simulink model "Multiuav"  (Simulink 4.00)
settings: Solver=FixedStepDiscrete  StartTime=0.0  StopTime=g_StopTime  FixedStep=g_SampleTime  RelTol=1e-3
undefined symbols (not defined in the file): ATRFunctions, g_AssignmentAlgorithm, g_CommandTurnRadius, g_CoordinationDelayDen, g_DefaultWaypointAltitude, g_EnableTarget, g_EnableVehicle, g_EntityTypes, g_MaxNumberTargets, g_MaxNumberVehicles, g_MaxReassignmentDeltaTime, g_ObjectMessageIDs, g_OptionSaveDataAVDS, g_OptionSaveDataPlot, g_SampleTime, g_SensorRollLimitDeg, g_TargetStates, g_Tasks, g_TypeAssignment, g_VehicleInputFiles, g_VehicleMemory, g_VehicleTypes, g_WaypointDefinitions, g_WaypointTypes
libraries: cooperative x42
(part 3 of 4)

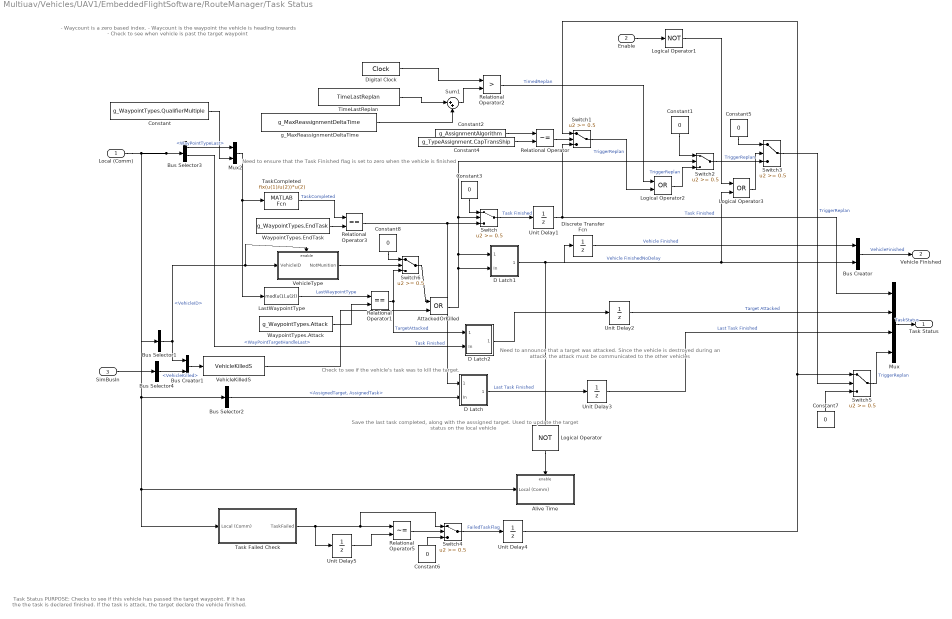
== system Multiuav/Vehicles/UAV1/EmbeddedFlightSoftware/RouteManager/Task Status ==
  note: - Waycount is a zero based index.
      | - Waycount is the waypoint the vehicle is
      | heading towards
      | - Check to see when vehicle is past the
      | target waypoint
  note: Need to ensure that the Task Finished
      | flag is set to zero when the vehicle is finished
  note: Check to see if the vehicle's
      | task was to kill the target.
  note: Need to announce that a target was
      | attacked. Since the vehicle is destroyed
      | during an attack, the attack must be
      | communicated to the other vehicles
  note: Save the last task completed,
      | along with the asssigned target.
      | Used to update the target status
      | on the local vehicle
  note: Task Status
      |
      | PURPOSE: Checks to see if this vehicle has passed the target waypoint. If it
      | has the the task is declared finished. If the task is attack, the target declare the
      | vehicle finished.
  Local (Comm) : Inport  Port=1  LatchInput=off  SampleTime=g_SampleTime
  Enable : Inport  Port=2  LatchInput=off  SampleTime=g_SampleTime
  SimBusIn : Inport  Port=3  LatchInput=off  SampleTime=g_SampleTime
  Alive Time : Subsystem  TreatAsAtomicUnit=on
      settings: RTWFcnNameOpts=Auto  RTWFileNameOpts=Auto
  AttackedOrKilled : Logic  Operator=OR  Inputs=2
  Bus Creator : BusCreator  Inputs=2
  Bus Creator1 : BusCreator  Inputs=2
  Bus Selector1 : BusSelector  OutputSignals=VehicleID  MuxedOutput=on
  Bus Selector2 : BusSelector  OutputSignals=Dynamics(com).TacticalManuevering.AssignedTarget,Dynamics(com).TacticalManuevering.AssignedTask  MuxedOutput=on
  Bus Selector3 : BusSelector  OutputSignals=Dynamics(com).TacticalManuevering.WayPointTypeLast,Dynamics(com).TacticalManuevering.WayPointTargetHandleLast  MuxedOutput=off
  Bus Selector4 : BusSelector  OutputSignals=ExternalTruth.VehicleKilled  MuxedOutput=on
  Constant : Constant  Value=g_WaypointTypes.QualifierMultiple
  Constant{1,3,5,8} (4 alike) : Constant  Orientation=down  Value=0
  Constant2 : Constant  Value=g_AssignmentAlgorithm
  Constant4 : Constant  Value=g_TypeAssignment.CapTransShip
  Constant6 : Constant  Orientation=up  Value=0
  Constant7 : Constant  Orientation=up  Value=0
  D Latch : Subsystem
      settings: RTWFcnNameOpts=Auto  RTWFileNameOpts=Auto
      mask Type: DLatch
      mask Description: D Latch Flip Flop Block
  D Latch1 : Subsystem
      settings: RTWFcnNameOpts=Auto  RTWFileNameOpts=Auto
      mask Type: DLatch
      mask Description: D Latch Flip Flop Block
  D Latch2 : Subsystem
      settings: RTWFcnNameOpts=Auto  RTWFileNameOpts=Auto
      mask Type: DLatch
      mask Description: D Latch Flip Flop Block
  Digital Clock : DigitalClock  SampleTime=g_SampleTime
  Discrete Transfer Fcn : DiscreteTransferFcn  Numerator=[1]  Denominator=[1 0 ]  SampleTime=g_SampleTime  Realization=auto
      settings: RTWStateStorageClass=Auto
  LastWaypointType : MATLABFcn  MATLABFcn=mod(u(1),u(2))  OutputDimensions=-1  OutputSignalType=auto  Output1D=on
  Logical Operator : Logic  Orientation=down  Operator=NOT  Inputs=2
  Logical Operator1 : Logic  Operator=NOT  Inputs=2
  Logical Operator2 : Logic  Operator=OR  Inputs=2
  Logical Operator3 : Logic  Operator=OR  Inputs=2
  Mux : Mux  Inputs=[1 1 2 1]
  Mux2 : Mux  Inputs=2
  Relational Operator : RelationalOperator  Operator=~=
  Relational Operator1 : RelationalOperator  Operator===
  Relational Operator2 : RelationalOperator  Operator=>
  Relational Operator3 : RelationalOperator  Operator===
  Relational Operator5 : RelationalOperator  Operator=~=
  Sum1 : Sum  Inputs=|++  SaturateOnIntegerOverflow=on
  Switch{,1..6} (7 alike) : Switch  Threshold=0.5
  Task Failed Check : Subsystem  TreatAsAtomicUnit=on
      settings: RTWFcnNameOpts=Auto  RTWFileNameOpts=Auto
  TaskCompleted : MATLABFcn  MATLABFcn=fix(u(1)/u(2))*u(2)  OutputDimensions=-1  OutputSignalType=auto  Output1D=on
  TimeLastReplan : DataStoreRead  DataStoreName=TimeLastReplan  SampleTime=g_SampleTime
  Unit Delay{1..5} (5 alike) : UnitDelay  X0=0  SampleTime=g_SampleTime
      settings: RTWStateStorageClass=Auto
  VehicleKilledS : S-Function  FunctionName=VehicleKilledS  Parameters=g_MaxNumberVehicles, g_MaxNumberTargets  PortCounts=[]  SFunctionModules=''
  VehicleType : Subsystem  TreatAsAtomicUnit=on
      settings: RTWFcnNameOpts=Auto  RTWFileNameOpts=Auto
  WaypointTypes.Attack : Constant  Value=g_WaypointTypes.Attack
  WaypointTypes.EndTask : Constant  Value=g_WaypointTypes.EndTask
  g_MaxReassignmentDeltaTime : Constant  Value=g_MaxReassignmentDeltaTime
  Task Status : Outport  Port=1
  Vehicle Finished : Outport  Port=2
  wires:
  Constant7/1 -> Switch5/3
  Switch5/1 -> Mux/4  "TriggerReplan"
  Unit Delay4/1 -> Switch5/1, Switch1/1
  Relational Operator2/1 -> Logical Operator2/1  "TimedReplan"
  Constant6/1 -> Switch4/3
  Switch4/1 -> Unit Delay4/1  "FailedTaskFlag"
  Unit Delay5/1 -> Relational Operator5/2
  Task Failed Check/1(TaskFailed) -> Switch4/1, Relational Operator5/1, Unit Delay5/1
  Local (Comm)/1 -> Task Failed Check/1(Local (Comm)), Alive Time/1(Local (Comm)), Bus Selector2/1, Bus Selector1/1, Bus Selector3/1
  WaypointTypes.EndTask/1 -> Relational Operator3/2
  WaypointTypes.Attack/1 -> Relational Operator1/2
  Constant3/1 -> Switch/1
  Switch/1 -> Unit Delay1/1  "Task Finished"
  Bus Selector2/1 -> D Latch/2(In)  "<AssignedTarget, AssignedTask>"
  Relational Operator3/1 -> D Latch/1(Enable), Switch/3  "Task Finished"
  Mux/1 -> Task Status/1  "TaskStatus"
  D Latch/1(Latched) -> Unit Delay3/1  "Last Task Finished"
  Discrete Transfer Fcn/1 -> Bus Creator/1  "Vehicle Finished"
  Unit Delay1/1 -> Switch1/3, Mux/1  "Task Finished"
  Unit Delay2/1 -> Mux/2  "Target Attacked"
  D Latch1/1(Latched) -> Discrete Transfer Fcn/1, Logical Operator/1, Bus Creator/2, Logical Operator3/2  "Vehicle FinishedNoDelay"
  Unit Delay3/1 -> Mux/3  "Last Task Finished"
  Bus Creator/1 -> Vehicle Finished/1  "VehicleFinished"
  Constant1/1 -> Switch2/1
  Logical Operator2/1 -> Switch2/3  "TriggerReplan"
  Bus Selector3/1 -> Mux2/1  "<WayPointTypeLast>"
  LastWaypointType/1 -> Relational Operator1/1  "LastWaypointType"
  TaskCompleted/1 -> Relational Operator3/1  "TaskCompleted"
  Constant/1 -> Mux2/2
  Mux2/1 -> LastWaypointType/1, TaskCompleted/1
  Bus Selector3/2 -> D Latch2/2(In)  "<WayPointTargetHandleLast>"
  D Latch2/1(Latched) -> Unit Delay2/1
  Logical Operator/1 -> Alive Time/Enable
  Relational Operator/1 -> Switch1/2
  Constant2/1 -> Relational Operator/1
  Constant4/1 -> Relational Operator/2
  Switch1/1 -> Logical Operator2/2  "TriggerReplan"
  Switch2/1 -> Switch3/3  "TriggerReplan"
  Relational Operator5/1 -> Switch4/2
  Sum1/1 -> Relational Operator2/2
  g_MaxReassignmentDeltaTime/1 -> Sum1/2
  TimeLastReplan/1 -> Sum1/1
  Digital Clock/1 -> Relational Operator2/1
  Constant5/1 -> Switch3/1
  Switch3/1 -> Switch5/2  "TriggerReplan"
  Logical Operator1/1 -> Logical Operator3/1
  Enable/1 -> Logical Operator1/1
  Logical Operator3/1 -> Switch3/2
  Bus Selector1/1 -> Bus Creator1/1, VehicleType/1(VehicleID), VehicleType/Enable  "<VehicleID>"
  Relational Operator1/1 -> Switch6/3, D Latch2/1(Enable)  "TargetAttacked"
  VehicleKilledS/1 -> AttackedOrKilled/2
  AttackedOrKilled/1 -> D Latch1/2(In), D Latch1/1(Enable), Switch2/2, Switch/2
  Bus Creator1/1 -> VehicleKilledS/1
  Bus Selector4/1 -> Bus Creator1/2  "<VehicleKilled>"
  SimBusIn/1 -> Bus Selector4/1
  Constant8/1 -> Switch6/1
  VehicleType/1(NotMunition) -> Switch6/2
  Switch6/1 -> AttackedOrKilled/1

== system Multiuav/Vehicles/UAV1/EmbeddedFlightSoftware/SensorManager/ATR Combined ==
  note: ATR Combined
      |
      | PURPOSE: Used to calculate a  combined ATR value for
      |      each target using single ATRs from this and other vehicles.
      |
      | IMPLEMENTATION:
      | - ATRCombined - calls the function "ATRFunctions" to calculate
      |      combined ATR values for the targets.
      | - Write ATR Memory - saves the last values of the single ATRs
      |       to enable a check for changes in these values.
  In1 : Inport  Port=1  LatchInput=off  SampleTime=g_SampleTime
  In2 : Inport  Port=2  LatchInput=off  SampleTime=g_SampleTime
  Enable : EnablePort
  ATRCombined : S-Function  FunctionName=ATRFunctionsCombinedS  Parameters=g_MaxNumberTargets  PortCounts=[]  SFunctionModules=''
  Bus Creator : BusCreator  Inputs=4
  Bus Creator1 : BusCreator  Inputs=4
  Demux : Demux  Outputs=[g_MaxNumberTargets,g_MaxNumberTargets,g_MaxNumberTargets,g_MaxNumberTargets,g_MaxNumberTargets,g_MaxNumberTargets]  BusSelectionMode=off
  Digital Clock : DigitalClock  SampleTime=g_SampleTime
  Write ATR Memory : DataStoreWrite  DataStoreName=ATRMemory  SampleTime=g_SampleTime
  Out1 : Outport  Port=1
  wires:
  Demux/6 -> Bus Creator1/4  "NumberValidHeadings"
  Demux/5 -> Bus Creator/4  "DesiredHeadings04"
  Demux/4 -> Bus Creator/3  "DesiredHeadings03"
  Demux/3 -> Bus Creator/2  "DesiredHeadings02"
  Demux/2 -> Bus Creator/1  "DesiredHeadings01"
  In1/1 -> ATRCombined/1
  In2/1 -> Write ATR Memory/1
  Digital Clock/1 -> Bus Creator1/1  "ATR Combined Time"
  Bus Creator1/1 -> Out1/1  "ATR Combined"
  Demux/1 -> Bus Creator1/2  "CombinedATRValues"
  Bus Creator/1 -> Bus Creator1/3  "Desired Headings"
  ATRCombined/1 -> Demux/1  "ATR Combined"

== system Multiuav/Vehicles/UAV1/EmbeddedFlightSoftware/SensorManager/ATR Single ==
  note: ATR Single
      |
      | PURPOSE: This block  is used to calculate a  value for ATR
      |      for a given target based on sensor data from this vehicle.
      |
      | IMPLEMENTATION:
      | - Automatic Target Recognition (ATR) - calls the M-function,
      |      "ATRFunctions" to calculation the single ATR value.
      | - Save Last Sensor Update - saves the last sensed values of the targets from
      |      the local vehicle to enable a check for changes in these values.
  VehicleID Psi SensedTargets : Inport  Port=1  LatchInput=off  SampleTime=g_SampleTime
  Target Truth : Inport  Port=2  LatchInput=off  SampleTime=g_SampleTime
  SendFlag : Inport  Port=3  LatchInput=off  SampleTime=g_SampleTime
  TargetStatus : Inport  Port=4  LatchInput=off  SampleTime=g_SampleTime
  Enable : EnablePort
  Bus Selector : BusSelector  OutputSignals=SensedTargets  MuxedOutput=off
  Save Last Sensor Update : DataStoreWrite  DataStoreName=LastSensorUpdate  SampleTime=g_SampleTime
  SingleATR : Subsystem  TreatAsAtomicUnit=on
      settings: RTWFcnNameOpts=Auto  RTWFileNameOpts=Auto
  ATR Single : Outport  Port=1
  wires:
  TargetStatus/1 -> SingleATR/3(TargetStatus)
  SendFlag/1 -> SingleATR/Enable
  Bus Selector/1 -> Save Last Sensor Update/1  "<SensedTargets>"
  Target Truth/1 -> SingleATR/2("Target Truth ")
  SingleATR/1(Out1) -> ATR Single/1
  VehicleID Psi SensedTargets/1 -> SingleATR/1(VehicleID Psi), Bus Selector/1

== system Multiuav/Vehicles/UAV1/EmbeddedFlightSoftware/SensorManager/BDA ==
  note: BDA
      |
      | PURPOSE: This block  is used to calculate a  value for BDA for a
      |      given target based on sensor data from this vehicle. The block "
      |
      | IMPLEMENTATION:
      | - BDA Calculation - calls the M-function, "ATRFunctions" to calculate
      |      a BDA value if it is appropriate to do so.
  VehicleID Psi SensedTargets : Inport  Port=1  LatchInput=off  SampleTime=g_SampleTime
  Target Truth : Inport  Port=2  LatchInput=off  SampleTime=g_SampleTime
  Local (Comm) : Inport  Port=3  LatchInput=off  SampleTime=g_SampleTime
  SimBusIn : Inport  Port=4  LatchInput=off  SampleTime=g_SampleTime
  Enable : EnablePort
  BDA Calculation : MATLABFcn  MATLABFcn=ATRFunctions('BDA',u)  OutputDimensions=g_MaxNumberTargets  OutputSignalType=auto  Output1D=on
  Bus Selector : BusSelector  OutputSignals=SensedTargets  MuxedOutput=off
  Bus Selector1 : BusSelector  OutputSignals=VehicleID,EFS(com).TargetManager(com).Target Status.TargetStatus  MuxedOutput=on
  Bus Selector2 : BusSelector  OutputSignals=ExternalTruth.TargetState  MuxedOutput=off
  Mux2 : Mux  Inputs=4
  BDA : Outport  Port=1
  wires:
  VehicleID Psi SensedTargets/1 -> Bus Selector/1
  Target Truth/1 -> Mux2/3
  Bus Selector/1 -> Mux2/2  "<SensedTargets>"
  Mux2/1 -> BDA Calculation/1
  Local (Comm)/1 -> Bus Selector1/1
  Bus Selector1/1 -> Mux2/1  "<VehicleID, TargetStatus>"
  SimBusIn/1 -> Bus Selector2/1
  Bus Selector2/1 -> Mux2/4  "<TargetState>"
  BDA Calculation/1 -> BDA/1  "BDA"

== system Multiuav/Vehicles/UAV1/EmbeddedFlightSoftware/TargetManager/New Target Check ==
  TargetStatus : Inport  Port=1  LatchInput=off
  And 1 : Logic  Operator=AND  Inputs=2
  And 3 : Logic  Operator=OR  Inputs=1
  Check for new target : RelationalOperator  Operator===
  Check for new target1 : RelationalOperator  Operator=~=
  Constant1 : Constant  Value=g_TargetStates.StateDetectedNotClassified*ones(g_MaxNumberTargets,1)
  No Alg Loop3 : UnitDelay  X0=0  SampleTime=g_SampleTime
      settings: RTWStateStorageClass=Auto
  New Target : Outport  Port=1
  wires:
  Constant1/1 -> Check for new target/1
  Check for new target1/1 -> And 1/2
  No Alg Loop3/1 -> Check for new target1/2
  And 3/1 -> New Target/1
  And 1/1 -> And 3/1
  TargetStatus/1 -> Check for new target/2, Check for new target1/1, No Alg Loop3/1
  Check for new target/1 -> And 1/1

== system Multiuav/Vehicles/UAV1/EmbeddedFlightSoftware/TargetManager/Sensed Target  Information ==
  In1 : Inport  Port=1  LatchInput=off
  Bus Creator : BusCreator  Inputs=1
  Bus Selector5 : BusSelector  OutputSignals=ExternalTruth.TargetState  MuxedOutput=off
  PreventLoopback : Gain  Gain=1  Multiplication=Element-wise(K.*u)  SaturateOnIntegerOverflow=on
  Out1 : Outport  Port=1
  wires:
  Bus Creator/1 -> Out1/1  "SensedTargetInformation"
  Bus Selector5/1 -> PreventLoopback/1  "<TargetState>"
  In1/1 -> Bus Selector5/1
  PreventLoopback/1 -> Bus Creator/1  "Targets"

== system Multiuav/Vehicles/UAV1/EmbeddedFlightSoftware/TargetManager/Target Status ==
  note: Target Status
      |
      | PURPOSE: This block is used to calculate and maintain the staus of each
      | of the targets. The block "Update Target Status" calls the
      | M-function "TargetStatus" to do the calculations.
      |
      |
      | IMPLEMENTATION:
      | - TargetStatusS - calls the MATLAB function "TargetStatus" to update the
      |      status of the targets.
      |
      | Target States:
      | 0 - Not Detected (~D)
      | 1 - Detected/Not Classified (D/~C)
      | 2 -  Classified/Not Attacked (C/~A)
      | 3 - Attacked/Not Killed (A/~K)
      | 4 - Killed/Not Verified (K/~V)
      | 5 - Verified  (V)
  Local (Comm) : Inport  Port=1  LatchInput=off  SampleTime=g_SampleTime
  Combined ATR : Inport  Port=2  LatchInput=off  SampleTime=g_SampleTime
  SimBusIn : Inport  Port=3  LatchInput=off  SampleTime=g_SampleTime
  ComBusIn : Inport  Port=4  LatchInput=off  SampleTime=g_SampleTime
  Enable : EnablePort
  Bus Selector : BusSelector  OutputSignals=VehicleID,Time,EFS(com).RouteManager(com).TaskStatus.Last Task Finished,EFS(com).SensorManager(com).ATR Combined.NumberValidHeadings  MuxedOutput=on
  Bus Selector1 : BusSelector  OutputSignals=TargetStatus,TargetAttacked  MuxedOutput=on
  Bus Selector4 : BusSelector  OutputSignals=ExternalTruth.VehicleIsDead  MuxedOutput=on
  Demux : Demux  Outputs=[g_MaxNumberTargets 1]  BusSelectionMode=off
  Mux2 : Mux  Inputs=3
  TargetStatusS : S-Function  FunctionName=TargetStatusS  Parameters=g_MaxNumberTargets,g_MaxNumberVehicles  PortCounts=[]  SFunctionModules=''
  "Write Last Combined ATR/BDA " : DataStoreWrite  DataStoreName=LastCombinedATR  SampleTime=g_SampleTime
  Write Last Vehicle Finished : DataStoreWrite  DataStoreName=LastVehicleFinished  SampleTime=g_SampleTime
  Target Status : Outport  Port=1
  Changed Status : Outport  Port=2
  wires:
  Demux/2 -> Changed Status/1  "TargetStatus02"
  SimBusIn/1 -> Bus Selector4/1
  Bus Selector4/1 -> Write Last Vehicle Finished/1  "<VehicleIsDead>"
  TargetStatusS/1 -> Demux/1  "TargetStatus"
  Demux/1 -> Target Status/1  "TargetStatus"
  Combined ATR/1 -> Mux2/2, "Write Last Combined ATR/BDA "/1
  ComBusIn/1 -> Bus Selector1/1
  Bus Selector/1 -> Mux2/1  "<VehicleID, Time, Last Task Finished, NumberValidHeadings>"
  Bus Selector1/1 -> Mux2/3  "<TargetStatus, TargetAttacked>"
  Local (Comm)/1 -> Bus Selector/1
  Mux2/1 -> TargetStatusS/1  "Target Manager"

== system Multiuav/Vehicles/UAV1/ReceiveTruth/ImplementNewAssignment/VehicleAlive ==
  In1 : Inport  Port=1  LatchInput=off
  In2 : Inport  Port=2  LatchInput=off
  Enable : EnablePort
  Bus Selector1 : BusSelector  OutputSignals=ChangeAssignmentFlagSelf  MuxedOutput=off
  Greater : Subsystem
      settings: RTWFcnNameOpts=Auto  RTWFileNameOpts=Auto
  NewAssignment : Subsystem  TreatAsAtomicUnit=on
      settings: RTWFcnNameOpts=Auto  RTWFileNameOpts=Auto
  Selector : Selector  InputType=Vector  ElementSrc=External  Elements=[1 3]  RowSrc=Internal  Rows=1  ColumnSrc=Internal  Columns=1  InputPortWidth=g_MaxNumberVehicles
  wires:
  Bus Selector1/1 -> Selector/1  "<ChangeAssignmentFlagSelf>"
  Selector/1 -> Greater/1(Signal)
  In1/1 -> NewAssignment/1(VehicleID), Selector/2
  Greater/1(Greater?) -> NewAssignment/Enable
  In2/1 -> Bus Selector1/1

== system Multiuav/Vehicles/UAV1/SendMessages/SendATRTime/Enabled Subsystem ==
  ATRTime : Inport  Port=1  LatchInput=off
  Enable : EnablePort
  Digital Clock : DigitalClock  SampleTime=g_SampleTime
  SaveWaypointIndex : DataStoreWrite  DataStoreName=ATRTime  SampleTime=g_SampleTime
  TimeStamp : Outport  Port=1
  wires:
  ATRTime/1 -> SaveWaypointIndex/1
  Digital Clock/1 -> TimeStamp/1

== system Multiuav/Vehicles/UAV1/SendMessages/SendAuctionData/Enabled Subsystem ==
  MessageNumber : Inport  Port=1  LatchInput=off
  Enable : EnablePort
  Data Store Write : DataStoreWrite  DataStoreName=LastMessageNumber  SampleTime=g_SampleTime
  Digital Clock : DigitalClock  SampleTime=g_SampleTime
  TimeStamp : Outport  Port=1
  wires:
  MessageNumber/1 -> Data Store Write/1
  Digital Clock/1 -> TimeStamp/1

== system Multiuav/Vehicles/UAV1/SendMessages/SendChangedStatus/Enabled Subsystem ==
  Enable : EnablePort
  Digital Clock : DigitalClock  SampleTime=g_SampleTime
  TimeStamp : Outport  Port=1
  wires:
  Digital Clock/1 -> TimeStamp/1

== system Multiuav/Vehicles/UAV1/SendMessages/SendPositionFlag/Enabled Subsystem ==
  PositionFlag : Inport  Port=1  LatchInput=off
  Enable : EnablePort
  Digital Clock : DigitalClock  SampleTime=g_SampleTime
  SaveWaypointIndex : DataStoreWrite  DataStoreName=PositionFlag  SampleTime=g_SampleTime
  TimeStamp : Outport  Port=1
  wires:
  Digital Clock/1 -> TimeStamp/1
  PositionFlag/1 -> SaveWaypointIndex/1

== system Multiuav/Vehicles/UAV1/SendMessages/SendPositionID/Enabled Subsystem ==
  PositionSendFlag Time : Inport  Port=1  LatchInput=off
  Enable : EnablePort
  Data Store Write : DataStoreWrite  DataStoreName=PositionsSendFlagTime  SampleTime=g_SampleTime
  Digital Clock : DigitalClock  SampleTime=g_SampleTime
  TimeStamp : Outport  Port=1
  wires:
  PositionSendFlag Time/1 -> Data Store Write/1
  Digital Clock/1 -> TimeStamp/1

== system Multiuav/Vehicles/UAV1/SendMessages/SendTargetAttacked/Enabled Subsystem ==
  "TargetAttacked " : Inport  Port=1  LatchInput=off
  Enable : EnablePort
  Digital Clock : DigitalClock  SampleTime=g_SampleTime
  SaveWaypointIndex : DataStoreWrite  DataStoreName=TargetAttacked  SampleTime=g_SampleTime
  TimeStamp : Outport  Port=1
  wires:
  Digital Clock/1 -> TimeStamp/1
  "TargetAttacked "/1 -> SaveWaypointIndex/1

== system Multiuav/Vehicles/UAV1/SendMessages/SendTargetStatus/Enabled Subsystem ==
  Enable : EnablePort
  Digital Clock : DigitalClock  SampleTime=g_SampleTime
  TimeStamp : Outport  Port=1
  wires:
  Digital Clock/1 -> TimeStamp/1

== system Multiuav/Vehicles/UAV1/SendMessages/SendTaskBenefits/Enabled Subsystem ==
  ReplanRound : Inport  Port=1  LatchInput=off
  Enable : EnablePort
  Data Store Write : DataStoreWrite  DataStoreName=LastReplanRound  SampleTime=g_SampleTime
  Digital Clock : DigitalClock  SampleTime=g_SampleTime
  TimeStamp : Outport  Port=1
  wires:
  ReplanRound/1 -> Data Store Write/1
  Digital Clock/1 -> TimeStamp/1

== system Multiuav/Vehicles/UAV1/SendMessages/SendTriggerReplan/Enabled Subsystem ==
  Enable : EnablePort
  Digital Clock : DigitalClock  SampleTime=g_SampleTime
  TimeStamp : Outport  Port=1
  wires:
  Digital Clock/1 -> TimeStamp/1

== system Multiuav/Vehicles/UAV1/SendMessages/SendWaypointNumber/Enabled Subsystem ==
  Waypoint : Inport  Port=1  LatchInput=off
  Enable : EnablePort
  Digital Clock : DigitalClock  SampleTime=g_SampleTime
  SaveWaypointIndex : DataStoreWrite  DataStoreName=WaypoinNumber  SampleTime=g_SampleTime
  TimeStamp : Outport  Port=1
  wires:
  Digital Clock/1 -> TimeStamp/1
  Waypoint/1 -> SaveWaypointIndex/1

== system Multiuav/Vehicles/UAV1/SendTruth/SendNewAssignment/Changed1 ==
  Signal : Inport  Port=1  LatchInput=off
  Relational Operator3 : RelationalOperator  Operator=>
  Unit Delay : UnitDelay  X0=0  SampleTime=g_SampleTime
      settings: RTWStateStorageClass=Auto
  Greater? : Outport  Port=1
  wires:
  Unit Delay/1 -> Relational Operator3/2
  Relational Operator3/1 -> Greater?/1
  Signal/1 -> Relational Operator3/1, Unit Delay/1

== system Multiuav/Vehicles/UAV1/SendTruth/SendNewAssignment/Enabled Subsystem ==
  Enable : EnablePort
  Digital Clock : DigitalClock  SampleTime=g_SampleTime
  TimeStamp : Outport  Port=1
  wires:
  Digital Clock/1 -> TimeStamp/1

== system Multiuav/Vehicles/UAV1/SendTruth/SendTargetStatus/Enabled Subsystem ==
  TargetStatus : Inport  Port=1  LatchInput=off
  Enable : EnablePort
  Data Store Write : DataStoreWrite  DataStoreName=TargetStatus  SampleTime=g_SampleTime
  Digital Clock : DigitalClock  SampleTime=g_SampleTime
  TimeStamp : Outport  Port=1
  wires:
  Digital Clock/1 -> TimeStamp/1
  TargetStatus/1 -> Data Store Write/1

== system Multiuav/Vehicles/UAV1/SendTruth/SendTrackList/Enabled Subsystem ==
  TrackList : Inport  Port=1  LatchInput=off
  Enable : EnablePort
  Data Store Write : DataStoreWrite  DataStoreName=TrackList  SampleTime=g_SampleTime
  Digital Clock : DigitalClock  SampleTime=g_SampleTime
  TimeStamp : Outport  Port=1
  wires:
  Digital Clock/1 -> TimeStamp/1
  TrackList/1 -> Data Store Write/1

== system Multiuav/Vehicles/UAV1/SendTruth/SendVehicleIsDead/Enabled Subsystem ==
  State : Inport  Port=1  LatchInput=off
  Enable : EnablePort
  Digital Clock : DigitalClock  SampleTime=g_SampleTime
  Save : DataStoreWrite  DataStoreName=VehicleIDead  SampleTime=g_SampleTime
  TimeStamp : Outport  Port=1
  wires:
  Digital Clock/1 -> TimeStamp/1
  State/1 -> Save/1

== system Multiuav/Vehicles/UAV1/SendTruth/SendWeaponsRelease/Enabled Subsystem ==
  WeaponID : Inport  Port=1  LatchInput=off
  Enable : EnablePort
  Data Store Write : DataStoreWrite  DataStoreName=WeaponID  SampleTime=g_SampleTime
  Digital Clock : DigitalClock  SampleTime=g_SampleTime
  TimeStamp : Outport  Port=1
  wires:
  WeaponID/1 -> Data Store Write/1
  Digital Clock/1 -> TimeStamp/1

== system Multiuav/Vehicles/UAV1/EmbeddedFlightSoftware/CooperationManager/Calculate Assignment/CapTransShip ==
  note: Calculate Assignment
      |
      | PURPOSE: Calculate the assignments for the vehicles based on the current
      |      state of the targets and vehicles.
      |
      | IMPLEMENTATION:
      | - CapTransShipIO - calculates the costs/bennefits associated with the vehicle
      |      task assignments. "CapTransShipIO" also formats the data into the input
      |      form expected by the assignment algorithm.
      | - Capacitative Transshipment Solver - this is an interface to a compiled S-function
      |      that implements a capacitated transhipment algorithm. It is used to select the
      |      target and task assignment for all of the vehicles.
      | - Assignment for Local Vehicle - uses the current vehicle's ID to select and output
      |      the target and task assignment for this vehicle.
  ComBusLocalIn : Inport  Port=1  LatchInput=off  SampleTime=g_SampleTime
  ComBusIn : Inport  Port=2  LatchInput=off  SampleTime=g_SampleTime
  Enable : EnablePort
  Assignment for Local Vehicle : Subsystem
      settings: RTWFcnNameOpts=Auto  RTWFileNameOpts=Auto
  Bus Selector1 : BusSelector  OutputSignals=VehicleID,EFS(com).TargetManager(com).Target Status.TargetStatus  MuxedOutput=on
  Bus Selector2 : BusSelector  OutputSignals=ETACostToSearch,TargetAttacked  MuxedOutput=on
  CapTransShipIOInS : S-Function  FunctionName=CapTransShipIOInS  Parameters=g_MaxNumberTargets,g_MaxNumberVehicles,g_Tasks.NumberTasks  PortCounts=[]  SFunctionModules=''
  Capacitative Transshipment Solver : S-Function  FunctionName=CapTranShipDll  Parameters=g_MaxNumberVehicles,g_MaxNumberTargets,g_Tasks.NumberTasks  PortCounts=[]  SFunctionModules=''
  Mux3 : Mux  Inputs=2
  Local Assignment : Outport  Port=1  InitialOutput=[0,0,0]
  wires:
  Assignment for Local Vehicle/1(Out1) -> Local Assignment/1
  ComBusIn/1 -> Bus Selector2/1
  CapTransShipIOInS/1 -> Capacitative Transshipment Solver/1
  Mux3/1 -> CapTransShipIOInS/1
  Capacitative Transshipment Solver/1 -> Assignment for Local Vehicle/2(In2)  "Assignment"
  Bus Selector1/1 -> Mux3/1  "<VehicleID, TargetStatus>"
  ComBusLocalIn/1 -> Bus Selector1/1, Assignment for Local Vehicle/1(In1)
  Bus Selector2/1 -> Mux3/2  "<ETACostToSearch, TargetAttacked>"

== system Multiuav/Vehicles/UAV1/EmbeddedFlightSoftware/CooperationManager/Calculate Assignment/DistAuctItCapTransShip ==
  ComBusLocalIn : Inport  Port=1  LatchInput=off  SampleTime=g_SampleTime
  ComBusIn : Inport  Port=2  LatchInput=off  SampleTime=g_SampleTime
  SimBusIn : Inport  Port=3  LatchInput=off  SampleTime=g_SampleTime
  EnableType : Inport  Port=4  LatchInput=off  SampleTime=g_SampleTime
  Enable : EnablePort
  Assignment Algorithm : Subsystem
      settings: RTWFcnNameOpts=Auto  RTWFileNameOpts=Auto
  Bus Creator : BusCreator  Inputs=2
  Message Processing : Subsystem
      settings: RTWFcnNameOpts=Auto  RTWFileNameOpts=Auto
  Not Used : Constant  Value=[0 0]
  Replan Logic : Subsystem
      settings: RTWFcnNameOpts=Auto  RTWFileNameOpts=Auto
  Store Benefits : Subsystem  TreatAsAtomicUnit=on
      settings: RTWFcnNameOpts=Auto  RTWFileNameOpts=Auto
  Local Assignment : Outport  Port=1
  AuctionData : Outport  Port=2
  wires:
  EnableType/1 -> Replan Logic/1(EnableType)
  Store Benefits/1(BenefitsStored) -> Assignment Algorithm/3(StoredBenefits)
  Assignment Algorithm/2(TargetStates) -> Store Benefits/3(TargetStates)
  Assignment Algorithm/3(StoreBenefits) -> Store Benefits/Enable
  Message Processing/1(NewBid) -> Assignment Algorithm/1(NewBid)
  Message Processing/2(NewAssignment) -> Assignment Algorithm/2(NewAssignment)
  Message Processing/3(RoundComplete) -> Assignment Algorithm/4(RoundComplete)
  Assignment Algorithm/1(AuctionData) -> AuctionData/1  "AuctionData"
  Replan Logic/1(ReplanTrigger) -> Assignment Algorithm/5(ReplanTrigger), Message Processing/4(ReplanTrigger)  "ReplanTrigger"
  ComBusLocalIn/1 -> Assignment Algorithm/6(CommBusLocalIn), Store Benefits/2(CommBusLocalIn), Message Processing/3(CommBusLocalIn)
  SimBusIn/1 -> Message Processing/2(SimBusIn)
  ComBusIn/1 -> Store Benefits/1(CommBusIn), Message Processing/1(CommBusIn)
  Not Used/1 -> Bus Creator/1
  Bus Creator/1 -> Local Assignment/1
  Assignment Algorithm/4(NewAssignmentTime) -> Bus Creator/2  "NewAssignmetTime"

== system Multiuav/Vehicles/UAV1/EmbeddedFlightSoftware/CooperationManager/Calculate Assignment/DistItCapTransShip ==
  ComBusLocalIn : Inport  Port=1  LatchInput=off  SampleTime=g_SampleTime
  ComBusIn : Inport  Port=2  LatchInput=off  SampleTime=g_SampleTime
  SimBusIn : Inport  Port=3  LatchInput=off  SampleTime=g_SampleTime
  EnableType : Inport  Port=4  LatchInput=off  SampleTime=g_SampleTime
  Enable : EnablePort
  Assignment Algorithm : Subsystem
      settings: RTWFcnNameOpts=Auto  RTWFileNameOpts=Auto
  Bus Creator : BusCreator  Inputs=2
  Demux : Demux  Outputs=7  BusSelectionMode=on
  Iteration Logic : Subsystem
      settings: RTWFcnNameOpts=Auto  RTWFileNameOpts=Auto
  Mux : Mux  Inputs=7
  Not Used : Constant  Value=[0 0]
  Replan Logic : Subsystem
      settings: RTWFcnNameOpts=Auto  RTWFileNameOpts=Auto
  Send Benefits : Subsystem  TreatAsAtomicUnit=on
      settings: RTWFcnNameOpts=Auto  RTWFileNameOpts=Auto
  Local Assignment : Outport  Port=1  InitialOutput=[0,0,0]
  Algorithm Data : Outport  Port=2
  wires:
  EnableType/1 -> Replan Logic/1(EnableType)
  Assignment Algorithm/3(SendBenefitsTrigger) -> Send Benefits/Enable
  Assignment Algorithm/1(TargetStatesOut) -> Send Benefits/3(TargetStates)
  Assignment Algorithm/2(ReplanRoundOut) -> Send Benefits/4(ReplanRound)
  Replan Logic/1(ReplanTrigger) -> Assignment Algorithm/8(ReplanTrigger)
  Demux/7 -> Assignment Algorithm/7(Sync)
  Demux/6 -> Assignment Algorithm/6(SearchBenefits)
  Demux/5 -> Assignment Algorithm/5(TimeToComplete)
  Demux/4 -> Assignment Algorithm/4(TaskBenefits)
  Demux/3 -> Assignment Algorithm/3(TargetStatesIn)
  Demux/2 -> Assignment Algorithm/2(ReplanRoundIn)
  Demux/1 -> Assignment Algorithm/1(ActiveVehicles)
  Mux/1 -> Demux/1
  Iteration Logic/7(Sync) -> Mux/7
  Iteration Logic/6(SearchBenefits) -> Mux/6
  Iteration Logic/5(TimeToComplete) -> Mux/5
  Iteration Logic/4(TaskBenefits) -> Mux/4
  Iteration Logic/3(TargetStates) -> Mux/3
  Iteration Logic/2(ReplanRound) -> Mux/2
  Iteration Logic/1(ActiveVehicles) -> Mux/1
  ComBusLocalIn/1 -> Assignment Algorithm/9(CommBusLocalIn), Send Benefits/2(CommBusLocalIn)
  SimBusIn/1 -> Iteration Logic/2(SimBusIn)
  ComBusIn/1 -> Send Benefits/1(CommBusIn), Iteration Logic/1(CommBusIn)
  Send Benefits/1(Algorithm Data) -> Algorithm Data/1
  Not Used/1 -> Bus Creator/1  "Localassignment"
  Bus Creator/1 -> Local Assignment/1
  Assignment Algorithm/4(NewAssignmentTime) -> Bus Creator/2  "NewAssignmentTime"

== system Multiuav/Vehicles/UAV1/EmbeddedFlightSoftware/CooperationManager/Calculate Assignment/ItCapTransShip ==
  note: ItCapTransShip
      |
      | PURPOSE: .
      |
      | IMPLEMENTATION:
      | - .
      | - .
      | - .
  ComBusLocalIn : Inport  Port=1  LatchInput=off  SampleTime=g_SampleTime
  ComBusIn : Inport  Port=2  LatchInput=off  SampleTime=g_SampleTime
  SimBusIn : Inport  Port=3  LatchInput=off  SampleTime=g_SampleTime
  Enable : EnablePort
  Bus Selector : BusSelector  OutputSignals=PositionID,WaypointIndex,TriggerReplan  MuxedOutput=on
  Bus Selector1 : BusSelector  OutputSignals=VehicleID,EFS(com).TargetManager(com).SensedTargetInformation.Targets,EFS(com).TargetManager(com).Target Status.TargetStatus,EFS(com).SensorManager(com).ATR Combined.Desired Headings.DesiredHeadings01,EFS(com).SensorManager(com).ATR Combined.Desired Headings.DesiredHeadings02,EFS(com).SensorManager(com).ATR Combined.Desired Headings.DesiredHeadings03,EFS(com).SensorManager(com).ATR Combined.Desired Headings.DesiredHeadings04,Dynamics(com).TacticalManuevering.CommandTurnRadius,Dynamics(com).TacticalManuevering.WayPointNumber,Dynamics(com).TacticalManuevering.WayPointTypeCurrent  MuxedOutput=on
  Bus Selector2 : BusSelector  OutputSignals=ExternalTruth.VehicleIsDead  MuxedOutput=on
  MultiTaskAssignIOS : S-Function  FunctionName=MultiTaskAssignIOS  Parameters=g_TypeAssignment.ItCapTransShip,g_MaxNumberTargets,g_MaxNumberVehicles  PortCounts=[]  SFunctionModules=''
  Mux : Mux  Inputs=3
  Local Assignment : Outport  Port=1  InitialOutput=[0,0,0]
  wires:
  Bus Selector2/1 -> Mux/2  "<VehicleIsDead>"
  SimBusIn/1 -> Bus Selector2/1
  Mux/1 -> MultiTaskAssignIOS/1
  Bus Selector1/1 -> Mux/3  "<VehicleID, Targets, TargetStatus, DesiredHeadings01, DesiredHeadings02, DesiredHeadings03, DesiredHeadings04, CommandTurnRadius, WayPointNumber, WayPointTypeCurrent>"
  Bus Selector/1 -> Mux/1  "<PositionID, WaypointIndex, TriggerReplan>"
  MultiTaskAssignIOS/1 -> Local Assignment/1
  ComBusIn/1 -> Bus Selector/1
  ComBusLocalIn/1 -> Bus Selector1/1

== system Multiuav/Vehicles/UAV1/EmbeddedFlightSoftware/CooperationManager/Calculate Assignment/ItJacobi ==
  note: ItCapTransShip
      |
      | PURPOSE: .
      |
      | IMPLEMENTATION:
      | - .
      | - .
      | - .
  ComBusLocalIn : Inport  Port=1  LatchInput=off  SampleTime=g_SampleTime
  ComBusIn : Inport  Port=2  LatchInput=off  SampleTime=g_SampleTime
  SimBusIn : Inport  Port=3  LatchInput=off  SampleTime=g_SampleTime
  Enable : EnablePort
  Bus Selector : BusSelector  OutputSignals=PositionID,WaypointIndex,TriggerReplan  MuxedOutput=on
  Bus Selector1 : BusSelector  OutputSignals=VehicleID,EFS(com).TargetManager(com).SensedTargetInformation.Targets,EFS(com).TargetManager(com).Target Status.TargetStatus,EFS(com).SensorManager(com).ATR Combined.Desired Headings.DesiredHeadings01,EFS(com).SensorManager(com).ATR Combined.Desired Headings.DesiredHeadings02,EFS(com).SensorManager(com).ATR Combined.Desired Headings.DesiredHeadings03,EFS(com).SensorManager(com).ATR Combined.Desired Headings.DesiredHeadings04,Dynamics(com).TacticalManuevering.CommandTurnRadius,Dynamics(com).TacticalManuevering.WayPointNumber,Dynamics(com).TacticalManuevering.WayPointTypeCurrent  MuxedOutput=on
  Bus Selector3 : BusSelector  OutputSignals=ExternalTruth.VehicleIsDead  MuxedOutput=on
  MultiTaskAssignIOS : S-Function  FunctionName=MultiTaskAssignIOS  Parameters=g_TypeAssignment.ItAuctionJacobi,g_MaxNumberTargets,g_MaxNumberVehicles  PortCounts=[]  SFunctionModules=''
  Mux : Mux  Inputs=3
  Local Assignment : Outport  Port=1  InitialOutput=[0,0,0]
  wires:
  Bus Selector3/1 -> Mux/2  "<VehicleIsDead>"
  SimBusIn/1 -> Bus Selector3/1
  Mux/1 -> MultiTaskAssignIOS/1
  Bus Selector1/1 -> Mux/3  "<VehicleID, Targets, TargetStatus, DesiredHeadings01, DesiredHeadings02, DesiredHeadings03, DesiredHeadings04, CommandTurnRadius, WayPointNumber, WayPointTypeCurrent>"
  Bus Selector/1 -> Mux/1  "<PositionID, WaypointIndex, TriggerReplan>"
  MultiTaskAssignIOS/1 -> Local Assignment/1
  ComBusIn/1 -> Bus Selector/1
  ComBusLocalIn/1 -> Bus Selector1/1

== system Multiuav/Vehicles/UAV1/EmbeddedFlightSoftware/CooperationManager/Calculate Assignment/MessageDisplay ==
  In1 : Inport  Port=1  LatchInput=off
  Enable : EnablePort
  MessageDisplayS : S-Function  Priority=1  FunctionName=MessageDisplayS  Parameters='Replan'  PortCounts=[]  SFunctionModules=''
  wires:
  In1/1 -> MessageDisplayS/1

== system Multiuav/Vehicles/UAV1/EmbeddedFlightSoftware/CooperationManager/Calculate Assignment/Relative Bennifits ==
  note: ItCapTransShip
      |
      | PURPOSE: .
      |
      | IMPLEMENTATION:
      | - .
      | - .
      | - .
  ComBusLocalIn : Inport  Port=1  LatchInput=off  SampleTime=g_SampleTime
  ComBusIn : Inport  Port=2  LatchInput=off  SampleTime=g_SampleTime
  SimBusIn : Inport  Port=3  LatchInput=off  SampleTime=g_SampleTime
  Enable : EnablePort
  Bus Selector1 : BusSelector  OutputSignals=VehicleID,EFS(com).TargetManager(com).SensedTargetInformation.Targets,EFS(com).TargetManager(com).Target Status.TargetStatus,EFS(com).SensorManager(com).ATR Combined.Desired Headings.DesiredHeadings01,EFS(com).SensorManager(com).ATR Combined.Desired Headings.DesiredHeadings02,EFS(com).SensorManager(com).ATR Combined.Desired Headings.DesiredHeadings03,EFS(com).SensorManager(com).ATR Combined.Desired Headings.DesiredHeadings04,Dynamics(com).TacticalManuevering.CommandTurnRadius,Dynamics(com).TacticalManuevering.WayPointNumber,Dynamics(com).TacticalManuevering.WayPointTypeCurrent  MuxedOutput=on
  Bus Selector3 : BusSelector  OutputSignals=PositionID,WaypointIndex,TriggerReplan  MuxedOutput=on
  Bus Selector4 : BusSelector  OutputSignals=ExternalTruth.VehicleIsDead  MuxedOutput=on
  MultiTaskAssignIOS : S-Function  FunctionName=MultiTaskAssignIOS  Parameters=g_TypeAssignment.RelativeBenefits,g_MaxNumberTargets,g_MaxNumberVehicles  PortCounts=[]  SFunctionModules=''
  Mux : Mux  Inputs=3
  Local Assignment : Outport  Port=1  InitialOutput=[0,0,0]
  wires:
  Bus Selector4/1 -> Mux/2  "<VehicleIsDead>"
  SimBusIn/1 -> Bus Selector4/1
  Mux/1 -> MultiTaskAssignIOS/1
  Bus Selector1/1 -> Mux/3  "<VehicleID, Targets, TargetStatus, DesiredHeadings01, DesiredHeadings02, DesiredHeadings03, DesiredHeadings04, CommandTurnRadius, WayPointNumber, WayPointTypeCurrent>"
  Bus Selector3/1 -> Mux/1  "<PositionID, WaypointIndex, TriggerReplan>"
  MultiTaskAssignIOS/1 -> Local Assignment/1
  ComBusIn/1 -> Bus Selector3/1
  ComBusLocalIn/1 -> Bus Selector1/1

== system Multiuav/Vehicles/UAV1/EmbeddedFlightSoftware/CooperationManager/Enable Reassignment/Assignment Time Delay ==
  note: Coordination Timing
      |
      | PURPOSE: This is a time delay to make sure that all of the
      |  other vehicle have had time to calculate the new
      |  routes. If they still have not the replan algorithm will
      |  not use that vehicle's old information.
  In : Inport  Port=1  LatchInput=off  SampleTime=g_SampleTime
  Discrete Transfer Fcn : DiscreteTransferFcn  Numerator=[1]  Denominator=g_CoordinationDelayDen  SampleTime=g_SampleTime  Realization=auto
      settings: RTWStateStorageClass=Auto
  InDelayed : Outport  Port=1
  wires:
  Discrete Transfer Fcn/1 -> InDelayed/1
  In/1 -> Discrete Transfer Fcn/1

== system Multiuav/Vehicles/UAV1/EmbeddedFlightSoftware/CooperationManager/Enable Reassignment/Changed ==
  Signal : Inport  Port=1  LatchInput=off
  Relational Operator3 : RelationalOperator  Operator=~=
  Unit Delay : UnitDelay  X0=0  SampleTime=g_SampleTime
      settings: RTWStateStorageClass=Auto
  Increased? : Outport  Port=1
  wires:
  Unit Delay/1 -> Relational Operator3/2
  Relational Operator3/1 -> Increased?/1
  Signal/1 -> Relational Operator3/1, Unit Delay/1

== system Multiuav/Vehicles/UAV1/EmbeddedFlightSoftware/CooperationManager/Enable Reassignment/Changed1 ==
  Signal : Inport  Port=1  LatchInput=off
  Relational Operator3 : RelationalOperator  Operator=~=
  Unit Delay : UnitDelay  X0=0  SampleTime=g_SampleTime
      settings: RTWStateStorageClass=Auto
  Changed? : Outport  Port=1
  wires:
  Unit Delay/1 -> Relational Operator3/2
  Relational Operator3/1 -> Changed?/1
  Signal/1 -> Relational Operator3/1, Unit Delay/1

== system Multiuav/Vehicles/UAV1/EmbeddedFlightSoftware/CooperationManager/Enable Reassignment/Changed2 ==
  Signal : Inport  Port=1  LatchInput=off
  Relational Operator3 : RelationalOperator  Operator=~=
  Unit Delay : UnitDelay  X0=0  SampleTime=g_SampleTime
      settings: RTWStateStorageClass=Auto
  Changed? : Outport  Port=1
  wires:
  Signal/1 -> Unit Delay/1, Relational Operator3/1
  Relational Operator3/1 -> Changed?/1
  Unit Delay/1 -> Relational Operator3/2

== system Multiuav/Vehicles/UAV1/EmbeddedFlightSoftware/CooperationManager/Task List/Update Task List ==
  note: Task List
  Vehicle ID : Inport  Port=1  LatchInput=off  SampleTime=g_SampleTime
  TargetStatus : Inport  Port=2  LatchInput=off  SampleTime=g_SampleTime
  Enable : EnablePort
  Mux : Mux  Inputs=2
  TargetStatusS : S-Function  FunctionName=TaskListS  Parameters=g_MaxNumberTargets  PortCounts=[]  SFunctionModules=''
  "Write Last Target Status " : DataStoreWrite  DataStoreName=LastTargetStatus  SampleTime=g_SampleTime
  UnassignedTaskFlag : Outport  Port=1
  wires:
  TargetStatusS/1 -> UnassignedTaskFlag/1
  Mux/1 -> TargetStatusS/1
  Vehicle ID/1 -> Mux/1
  TargetStatus/1 -> Mux/2, "Write Last Target Status "/1

== system Multiuav/Vehicles/UAV1/EmbeddedFlightSoftware/RouteManager/ReplanSingle/Replan ==
  note: RouteSelection
      |
      | PURPOSE: Calculates the ETA, cost and waypoint trajectory for the lowest
      |      cost flyable path to each of the targets, to accomplish the appropriate task,
      |      and stores the data for later use.
      |
      | Implementation:
      | - ReplanRoutes- calls the function, "ReplanRoutes" to do the calculations. The
      |      lowest cost set of waypoints for each known target is stored in the appropriate
      |      location in the global structure "VehicleMemory.RouteManager".
  In1 : Inport  Port=1  LatchInput=off
  Enable : EnablePort
  Bus Creator : BusCreator  Inputs=4
  Bus Selector : BusSelector  OutputSignals=Local Bus.VehicleID,Vehicle (Sim).EFS(sim).RouteManager(sim).VehicleFinished.Vehicle Finished,Local Bus.Dynamics(com).TacticalManuevering.CommandTurnRadius,Local Bus.Dynamics(com).AC Dynamics.Position_x,Local Bus.Dynamics(com).AC Dynamics.Position_y,Local Bus.Dynamics(com).AC Dynamics.Altitude,Local Bus.Dynamics(com).AC Dynamics.Psi,Local Bus.Dynamics(com).AC Dynamics.V North,Local Bus.Dynamics(com).AC Dynamics.V East,Local Bus.Dynamics(com).TacticalManuevering.CommandVelocity,Local Bus.Dynamics(com).TacticalManuevering.WayPointNumber,Local Bus.EFS(com).RouteManager(com).TaskStatus.Task Finished,Local Bus.EFS(com).TargetManager(com).Target Status.TargetStatus,Local Bus.EFS(com).SensorManager(com).ATR Combined.Desired Headings,TargetState  MuxedOutput=on
  Demux : Demux  Outputs=[g_MaxNumberTargets,g_MaxNumberTargets,g_MaxNumberTargets]  BusSelectionMode=off
  Digital Clock : DigitalClock  SampleTime=g_SampleTime
  ReplanRoutes : S-Function  FunctionName=ReplanRoutesS  Parameters=g_MaxNumberTargets  PortCounts=[]  SFunctionModules=''
  ReplanETAsCosts : Outport  Port=1
  wires:
  Demux/2 -> Bus Creator/3  "TargetETAs"
  Digital Clock/1 -> Bus Creator/1  "ReplanTime"
  In1/1 -> Bus Selector/1
  Bus Selector/1 -> ReplanRoutes/1  "<VehicleID, Vehicle Finished, CommandTurnRadius, Position_x, Position_y, Altitude, Psi, V North, V East, CommandVelocity, WayPointNumber, Task Finished, TargetStatus, Desired Headings, TargetState>"
  Demux/3 -> Bus Creator/4  "TargetToSearchDist"
  Bus Creator/1 -> ReplanETAsCosts/1  "Replan ETAs and Costs"
  ReplanRoutes/1 -> Demux/1
  Demux/1 -> Bus Creator/2  "TargetCosts"

== system Multiuav/Vehicles/UAV1/EmbeddedFlightSoftware/RouteManager/ReplanSingle/RouteSelection ==
  note: RouteSelection
      |
      | PURPOSE: This manager implements waypoints for the route selected for this
      | vehicle during the vehicle/target assignment in the cooperation manager.
      |
      | Implementation:
      | - RouteSelection - calls the function "RouteSelection" to implement waypoints
      |      for the route selected.
  In1 : Inport  Port=1  LatchInput=off
  Enable : EnablePort
  RouteSelection : S-Function  FunctionName=RouteSelectionS  PortCounts=[]  SFunctionModules=''
  wires:
  In1/1 -> RouteSelection/1

== system Multiuav/Vehicles/UAV1/EmbeddedFlightSoftware/RouteManager/Task Status/Alive Time ==
  Local (Comm) : Inport  Port=1  LatchInput=off  SampleTime=g_SampleTime
  Enable : EnablePort
  Bus Selector4 : BusSelector  OutputSignals=VehicleID  MuxedOutput=off
  Digital Clock : DigitalClock  SampleTime=g_SampleTime
  Mux : Mux  Inputs=2
  S-Function : S-Function  FunctionName=MonteCarloMetricS  Parameters='AliveTimeSeconds'  PortCounts=[]  SFunctionModules=''
  wires:
  Bus Selector4/1 -> Mux/1  "<VehicleID>"
  Local (Comm)/1 -> Bus Selector4/1
  Mux/1 -> S-Function/1
  Digital Clock/1 -> Mux/2

== system Multiuav/Vehicles/UAV1/EmbeddedFlightSoftware/RouteManager/Task Status/D Latch ==
  Enable : Inport  Orientation=down  Port=1  LatchInput=off
  In : Inport  Port=2  LatchInput=off  SampleTime=g_SampleTime
  D Latch : Subsystem  TreatAsAtomicUnit=on
      settings: RTWFcnNameOpts=Auto  RTWFileNameOpts=Auto
  Latched : Outport  Port=1  InitialOutput=0
  wires:
  Enable/1 -> D Latch/Enable
  D Latch/1(Q) -> Latched/1
  In/1 -> D Latch/1(D)

== system Multiuav/Vehicles/UAV1/EmbeddedFlightSoftware/RouteManager/Task Status/D Latch1 ==
  Enable : Inport  Orientation=down  Port=1  LatchInput=off
  In : Inport  Port=2  LatchInput=off  SampleTime=g_SampleTime
  D Latch : Subsystem  TreatAsAtomicUnit=on
      settings: RTWFcnNameOpts=Auto  RTWFileNameOpts=Auto
  Latched : Outport  Port=1  InitialOutput=0
  wires:
  In/1 -> D Latch/1(D)
  D Latch/1(Q) -> Latched/1
  Enable/1 -> D Latch/Enable

== system Multiuav/Vehicles/UAV1/EmbeddedFlightSoftware/RouteManager/Task Status/D Latch2 ==
  Enable : Inport  Orientation=down  Port=1  LatchInput=off
  In : Inport  Port=2  LatchInput=off  SampleTime=g_SampleTime
  D Latch : Subsystem  TreatAsAtomicUnit=on
      settings: RTWFcnNameOpts=Auto  RTWFileNameOpts=Auto
  Latched : Outport  Port=1  InitialOutput=0
  wires:
  Enable/1 -> D Latch/Enable
  D Latch/1(Q) -> Latched/1
  In/1 -> D Latch/1(D)

== system Multiuav/Vehicles/UAV1/EmbeddedFlightSoftware/RouteManager/Task Status/Task Failed Check ==
  Local (Comm) : Inport  Port=1  LatchInput=off
  Bus Selector1 : BusSelector  OutputSignals=Dynamics(com).TacticalManuevering.WayPointTypeCurrent,EFS(com).TargetManager(com).Target Status.TargetStatus  MuxedOutput=off
  Create Last Task : DataStoreMemory  DataStoreName=LastWaypointType  InitialValue=0
  Create Last Task1 : DataStoreMemory  DataStoreName=LastTargetState  InitialValue=g_TargetStates.StateUndefined*ones(g_MaxNumberTargets,1)
  Logical Operator : Logic  Operator=OR  Inputs=2
  Read Last Task : DataStoreRead  DataStoreName=LastWaypointType  SampleTime=g_SampleTime
  Read Last Task1 : DataStoreRead  DataStoreName=LastTargetState  SampleTime=g_SampleTime
  Relational Operator1 : RelationalOperator  Operator=~=
  Relational Operator4 : RelationalOperator  Operator=~=
  Task Failed Check : Subsystem  TreatAsAtomicUnit=on
      settings: RTWFcnNameOpts=Auto  RTWFileNameOpts=Auto
  TaskFailed : Outport  Port=1
  wires:
  Relational Operator1/1 -> Logical Operator/2
  Read Last Task1/1 -> Task Failed Check/2(LastTargetState), Relational Operator1/2
  Bus Selector1/2 -> Relational Operator1/1  "<TargetStatus>"
  Relational Operator4/1 -> Logical Operator/1
  Logical Operator/1 -> Task Failed Check/Enable
  Task Failed Check/1(TaskFailed) -> TaskFailed/1
  Bus Selector1/1 -> Relational Operator4/2  "<WayPointTypeCurrent>"
  Read Last Task/1 -> Relational Operator4/1
  Local (Comm)/1 -> Task Failed Check/1(Local (Comm)), Bus Selector1/1

== system Multiuav/Vehicles/UAV1/EmbeddedFlightSoftware/RouteManager/Task Status/VehicleType ==
  VehicleID : Inport  Port=1  LatchInput=off
  Enable : EnablePort
  EntityType : MATLABFcn  MATLABFcn=g_VehicleTypes(g_VehicleMemory(u).VehicleType).EntityType  OutputDimensions=-1  OutputSignalType=auto  Output1D=on
  Relational Operator4 : RelationalOperator  Operator=~=
  WaypointTypes.EndTask1 : Constant  Value=g_EntityTypes.Munition
  NotMunition : Outport  Port=1  InitialOutput=0
  wires:
  WaypointTypes.EndTask1/1 -> Relational Operator4/2
  EntityType/1 -> Relational Operator4/1  "TaskCompleted"
  VehicleID/1 -> EntityType/1
  Relational Operator4/1 -> NotMunition/1  "NotMunition"

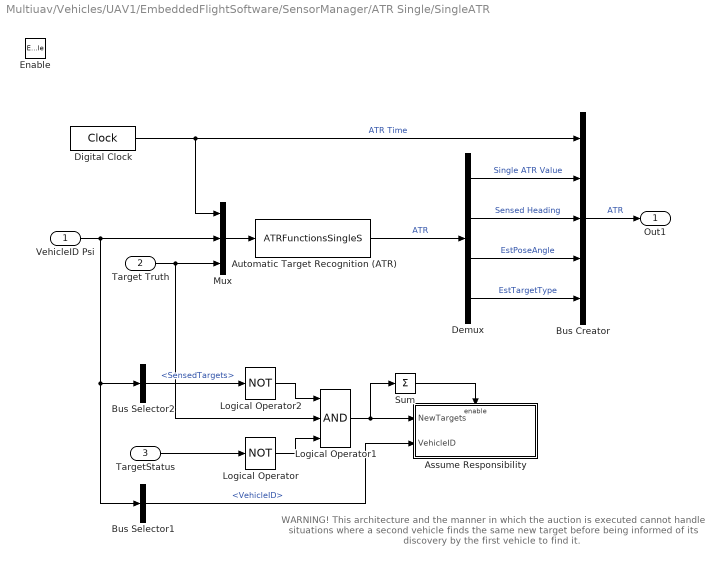
== system Multiuav/Vehicles/UAV1/EmbeddedFlightSoftware/SensorManager/ATR Single/SingleATR ==
  note: WARNING!
      | This architecture and the manner in which
      | the auction is executed cannot handle
      | situations where a second vehicle finds the
      | same new target before being informed of its
      | discovery by the first vehicle to find it.
  VehicleID Psi : Inport  Port=1  LatchInput=off
  "Target Truth " : Inport  Port=2  LatchInput=off
  TargetStatus : Inport  Port=3  LatchInput=off  SampleTime=g_SampleTime
  Enable : EnablePort
  Assume Responsibility : Subsystem  TreatAsAtomicUnit=on
      settings: RTWFcnNameOpts=Auto  RTWFileNameOpts=Auto
  Automatic Target Recognition (ATR) : S-Function  FunctionName=ATRFunctionsSingleS  Parameters=g_MaxNumberTargets  PortCounts=[]  SFunctionModules=''
  Bus Creator : BusCreator  Inputs=5
  Bus Selector1 : BusSelector  OutputSignals=VehicleID  MuxedOutput=off
  Bus Selector2 : BusSelector  OutputSignals=SensedTargets  MuxedOutput=off
  Demux : Demux  Outputs=[g_MaxNumberTargets,g_MaxNumberTargets,g_MaxNumberTargets,g_MaxNumberTargets]  BusSelectionMode=off
  Digital Clock : DigitalClock  SampleTime=g_SampleTime
  Logical Operator : Logic  Operator=NOT  Inputs=1
  Logical Operator1 : Logic  Operator=AND  Inputs=3
  Logical Operator2 : Logic  Operator=NOT  Inputs=1
  Mux : Mux  Inputs=3
  Sum : Sum  Inputs=+  SaturateOnIntegerOverflow=on
  Out1 : Outport  Port=1
  wires:
  Logical Operator2/1 -> Logical Operator1/1
  Bus Selector2/1 -> Logical Operator2/1  "<SensedTargets>"
  TargetStatus/1 -> Logical Operator/1
  Sum/1 -> Assume Responsibility/Enable
  Bus Selector1/1 -> Assume Responsibility/2(VehicleID)  "<VehicleID>"
  Logical Operator1/1 -> Assume Responsibility/1(NewTargets), Sum/1
  Logical Operator/1 -> Logical Operator1/3
  Demux/4 -> Bus Creator/5  "EstTargetType"
  Automatic Target Recognition (ATR)/1 -> Demux/1  "ATR"
  Demux/3 -> Bus Creator/4  "EstPoseAngle"
  Demux/2 -> Bus Creator/3  "Sensed Heading"
  "Target Truth "/1 -> Logical Operator1/2, Mux/3
  Bus Creator/1 -> Out1/1  "ATR"
  VehicleID Psi/1 -> Bus Selector2/1, Bus Selector1/1, Mux/2
  Mux/1 -> Automatic Target Recognition (ATR)/1
  Demux/1 -> Bus Creator/2  "Single ATR Value"
  Digital Clock/1 -> Mux/1, Bus Creator/1  "ATR Time"

== system Multiuav/Vehicles/UAV1/ReceiveTruth/ImplementNewAssignment/VehicleAlive/Greater ==
  Signal : Inport  Port=1  LatchInput=off
  Relational Operator3 : RelationalOperator  Operator=>
  Unit Delay : UnitDelay  X0=0  SampleTime=g_SampleTime
      settings: RTWStateStorageClass=Auto
  Greater? : Outport  Port=1
  wires:
  Unit Delay/1 -> Relational Operator3/2
  Relational Operator3/1 -> Greater?/1
  Signal/1 -> Relational Operator3/1, Unit Delay/1

== system Multiuav/Vehicles/UAV1/ReceiveTruth/ImplementNewAssignment/VehicleAlive/NewAssignment ==
  VehicleID : Inport  Port=1  LatchInput=off
  Enable : EnablePort
  ImplementNewAssignment : S-Function  FunctionName=ImplementNewAssignmentS  PortCounts=[]  SFunctionModules=''
  wires:
  VehicleID/1 -> ImplementNewAssignment/1
